simulink model "demonstrator"  (R2021a)
settings: Solver=VariableStepAuto  StartTime=0.0  StopTime=4000/3.2e6  RelTol=1e-3
values from neighbouring files (symbols this model uses):
  f_system = 64e6    (= 64000000)    [setup_demonstrator.m]
  fir_bbuf = reshape([fir_barker_13; fir_barker_13; fir_barker_13], [1, length(fir_barker_13)*3])    [setup_demonstrator.m]
  tx_data = [tx_data mbuf]    [setup_demonstrator.m]
undefined symbols (not defined in the file or in its folder): AXI4, designMultirateFIR, fsystem, Lite, xlfda_numerator
libraries: hdlBasic x533, hdlsllib x35, hdlDSPIP x21, hdlSSR x18, dspmlti4 x14, dspswit3 x8, dspsigops x5, vmcUtilities x4, hdlUtilities x4, simulink x3, dspsigattribs x2, commrandsrc3 x1
(part 9 of 10)

== system demonstrator/Receiver/Carrier Synchronisation/Generate Angle Error/Circular CORDIC/Vectoring Cell 1 ==
  x in : Inport
  y in : Inport  Port=2
  z in : Inport  Port=3
  AddSub1 : hdlBasic/AddSub  mode=Addition or Subtraction  use_carryin=off  use_carryout=off  en=off  latency=0  precision=User Defined  arith_type="Signed  (2's comp)"  n_bits=20  bin_pt=18  quantization=Truncate  overflow=Wrap  use_behavioral_HDL=on  hw_selection=Fabric  pipelined=off  use_rpm=on  XmcBlockStatus=1  maskContainerNames=tabcontainer1  block_type=addsub  block_config=sysgen:Addsub_config
  AddSub2 : hdlBasic/AddSub  mode=Addition or Subtraction  use_carryin=off  use_carryout=off  en=off  latency=0  precision=User Defined  arith_type="Signed  (2's comp)"  n_bits=15  bin_pt=12  quantization=Truncate  overflow=Wrap  use_behavioral_HDL=on  hw_selection=Fabric  pipelined=off  use_rpm=on  XmcBlockStatus=1  maskContainerNames=tabcontainer1  block_type=addsub  block_config=sysgen:Addsub_config
  AddSub3 : hdlBasic/AddSub  mode=Addition or Subtraction  use_carryin=off  use_carryout=off  en=off  latency=0  precision=User Defined  arith_type="Signed  (2's comp)"  n_bits=15  bin_pt=12  quantization=Truncate  overflow=Wrap  use_behavioral_HDL=on  hw_selection=Fabric  pipelined=off  use_rpm=on  XmcBlockStatus=1  maskContainerNames=tabcontainer1  block_type=addsub  block_config=sysgen:Addsub_config
  Constant : hdlBasic/Constant  const=atan(2^-i)  gui_display_data_type=Fixed-point  arith_type=Signed (2's comp)  n_bits=20  bin_pt=18  preci_type=Single  exp_width=8  frac_width=24  explicit_period=off  period=1  XmcBlockStatus=1  maskContainerNames=tabcontainer1  block_type=constant  block_config=sysgen:Constant_config
  Inverter : hdlBasic/Inverter  en=off  latency=0  XmcBlockStatus=1  maskContainerNames=group2  block_type=inv  block_config=sysgen:Inverter_config
  Logical : hdlBasic/Logical  logical_function=XOR  inputs=2  en=off  latency=0  precision=Full  arith_type=Unsigned  n_bits=1  bin_pt=0  align_bp=on  overflow=[]  quantization=[]  XmcBlockStatus=1  maskContainerNames=tabcontainer1  block_type=logical  block_config=sysgen:Logical_config
  Shift : hdlBasic/Shift  shift_dir=Right  shift_bits=i  en=off  latency=0  precision=User Defined  arith_type="Signed  (2's comp)"  n_bits=15  bin_pt=12  quantization=Truncate  overflow=Wrap  XmcBlockStatus=1  maskContainerNames=group2  block_type=shift  block_config=sysgen:Shift_config
  Shift1 : hdlBasic/Shift  shift_dir=Right  shift_bits=i  en=off  latency=0  precision=User Defined  arith_type="Signed  (2's comp)"  n_bits=15  bin_pt=12  quantization=Truncate  overflow=Wrap  XmcBlockStatus=1  maskContainerNames=group2  block_type=shift  block_config=sysgen:Shift_config
  Slice : hdlBasic/Slice  nbits=1  boolean_output=on  mode=Upper Bit Location + Width  bit1=0  base1=MSB of Input  bit0=0  base0=LSB of Input  XmcBlockStatus=1  maskContainerNames=group1  block_type=slice  block_config=sysgen:Slice_config
  Slice1 : hdlBasic/Slice  nbits=1  boolean_output=on  mode=Upper Bit Location + Width  bit1=0  base1=MSB of Input  bit0=0  base0=LSB of Input  XmcBlockStatus=1  maskContainerNames=group1  block_type=slice  block_config=sysgen:Slice_config
  x out : Outport  VectorParamsAs1DForOutWhenUnconnected=off
  y out : Outport  Port=2  VectorParamsAs1DForOutWhenUnconnected=off
  z out : Outport  Port=3  VectorParamsAs1DForOutWhenUnconnected=off
  wires:
  AddSub1/1 -> z out/1
  Constant/1 -> AddSub1/2
  z in/1 -> AddSub1/1
  AddSub3/1 -> y out/1
  AddSub2/1 -> x out/1
  Inverter/1 -> AddSub3/3
  Shift/1 -> AddSub3/2
  Shift1/1 -> AddSub2/2
  Logical/1 -> AddSub1/3, AddSub2/3, Inverter/1
  Slice1/1 -> Logical/2
  Slice/1 -> Logical/1
  y in/1 -> Slice1/1, Shift1/1, AddSub3/1
  x in/1 -> Slice/1, Shift/1, AddSub2/1

== system demonstrator/Receiver/Carrier Synchronisation/Generate Angle Error/Circular CORDIC/Vectoring Cell 2 ==
  x in : Inport
  y in : Inport  Port=2
  z in : Inport  Port=3
  AddSub1 : hdlBasic/AddSub  mode=Addition or Subtraction  use_carryin=off  use_carryout=off  en=off  latency=0  precision=User Defined  arith_type="Signed  (2's comp)"  n_bits=20  bin_pt=18  quantization=Truncate  overflow=Wrap  use_behavioral_HDL=on  hw_selection=Fabric  pipelined=off  use_rpm=on  XmcBlockStatus=1  maskContainerNames=tabcontainer1  block_type=addsub  block_config=sysgen:Addsub_config
  AddSub2 : hdlBasic/AddSub  mode=Addition or Subtraction  use_carryin=off  use_carryout=off  en=off  latency=0  precision=User Defined  arith_type="Signed  (2's comp)"  n_bits=15  bin_pt=12  quantization=Truncate  overflow=Wrap  use_behavioral_HDL=on  hw_selection=Fabric  pipelined=off  use_rpm=on  XmcBlockStatus=1  maskContainerNames=tabcontainer1  block_type=addsub  block_config=sysgen:Addsub_config
  AddSub3 : hdlBasic/AddSub  mode=Addition or Subtraction  use_carryin=off  use_carryout=off  en=off  latency=0  precision=User Defined  arith_type="Signed  (2's comp)"  n_bits=15  bin_pt=12  quantization=Truncate  overflow=Wrap  use_behavioral_HDL=on  hw_selection=Fabric  pipelined=off  use_rpm=on  XmcBlockStatus=1  maskContainerNames=tabcontainer1  block_type=addsub  block_config=sysgen:Addsub_config
  Constant : hdlBasic/Constant  const=atan(2^-i)  gui_display_data_type=Fixed-point  arith_type=Signed (2's comp)  n_bits=20  bin_pt=18  preci_type=Single  exp_width=8  frac_width=24  explicit_period=off  period=1  XmcBlockStatus=1  maskContainerNames=tabcontainer1  block_type=constant  block_config=sysgen:Constant_config
  Inverter : hdlBasic/Inverter  en=off  latency=0  XmcBlockStatus=1  maskContainerNames=group2  block_type=inv  block_config=sysgen:Inverter_config
  Logical : hdlBasic/Logical  logical_function=XOR  inputs=2  en=off  latency=0  precision=Full  arith_type=Unsigned  n_bits=1  bin_pt=0  align_bp=on  overflow=[]  quantization=[]  XmcBlockStatus=1  maskContainerNames=tabcontainer1  block_type=logical  block_config=sysgen:Logical_config
  Shift : hdlBasic/Shift  shift_dir=Right  shift_bits=i  en=off  latency=0  precision=User Defined  arith_type="Signed  (2's comp)"  n_bits=15  bin_pt=12  quantization=Truncate  overflow=Wrap  XmcBlockStatus=1  maskContainerNames=group2  block_type=shift  block_config=sysgen:Shift_config
  Shift1 : hdlBasic/Shift  shift_dir=Right  shift_bits=i  en=off  latency=0  precision=User Defined  arith_type="Signed  (2's comp)"  n_bits=15  bin_pt=12  quantization=Truncate  overflow=Wrap  XmcBlockStatus=1  maskContainerNames=group2  block_type=shift  block_config=sysgen:Shift_config
  Slice : hdlBasic/Slice  nbits=1  boolean_output=on  mode=Upper Bit Location + Width  bit1=0  base1=MSB of Input  bit0=0  base0=LSB of Input  XmcBlockStatus=1  maskContainerNames=group1  block_type=slice  block_config=sysgen:Slice_config
  Slice1 : hdlBasic/Slice  nbits=1  boolean_output=on  mode=Upper Bit Location + Width  bit1=0  base1=MSB of Input  bit0=0  base0=LSB of Input  XmcBlockStatus=1  maskContainerNames=group1  block_type=slice  block_config=sysgen:Slice_config
  x out : Outport  VectorParamsAs1DForOutWhenUnconnected=off
  y out : Outport  Port=2  VectorParamsAs1DForOutWhenUnconnected=off
  z out : Outport  Port=3  VectorParamsAs1DForOutWhenUnconnected=off
  wires:
  x in/1 -> AddSub2/1, Shift/1, Slice/1
  y in/1 -> AddSub3/1, Shift1/1, Slice1/1
  Slice/1 -> Logical/1
  Slice1/1 -> Logical/2
  Logical/1 -> Inverter/1, AddSub2/3, AddSub1/3
  Shift1/1 -> AddSub2/2
  Shift/1 -> AddSub3/2
  Inverter/1 -> AddSub3/3
  AddSub2/1 -> x out/1
  AddSub3/1 -> y out/1
  z in/1 -> AddSub1/1
  Constant/1 -> AddSub1/2
  AddSub1/1 -> z out/1

== system demonstrator/Receiver/Carrier Synchronisation/Generate Angle Error/Circular CORDIC/Vectoring Cell 3 ==
  x in : Inport
  y in : Inport  Port=2
  z in : Inport  Port=3
  AddSub1 : hdlBasic/AddSub  mode=Addition or Subtraction  use_carryin=off  use_carryout=off  en=off  latency=0  precision=User Defined  arith_type="Signed  (2's comp)"  n_bits=20  bin_pt=18  quantization=Truncate  overflow=Wrap  use_behavioral_HDL=on  hw_selection=Fabric  pipelined=off  use_rpm=on  XmcBlockStatus=1  maskContainerNames=tabcontainer1  block_type=addsub  block_config=sysgen:Addsub_config
  AddSub2 : hdlBasic/AddSub  mode=Addition or Subtraction  use_carryin=off  use_carryout=off  en=off  latency=0  precision=User Defined  arith_type="Signed  (2's comp)"  n_bits=15  bin_pt=12  quantization=Truncate  overflow=Wrap  use_behavioral_HDL=on  hw_selection=Fabric  pipelined=off  use_rpm=on  XmcBlockStatus=1  maskContainerNames=tabcontainer1  block_type=addsub  block_config=sysgen:Addsub_config
  AddSub3 : hdlBasic/AddSub  mode=Addition or Subtraction  use_carryin=off  use_carryout=off  en=off  latency=0  precision=User Defined  arith_type="Signed  (2's comp)"  n_bits=15  bin_pt=12  quantization=Truncate  overflow=Wrap  use_behavioral_HDL=on  hw_selection=Fabric  pipelined=off  use_rpm=on  XmcBlockStatus=1  maskContainerNames=tabcontainer1  block_type=addsub  block_config=sysgen:Addsub_config
  Constant : hdlBasic/Constant  const=atan(2^-i)  gui_display_data_type=Fixed-point  arith_type=Signed (2's comp)  n_bits=20  bin_pt=18  preci_type=Single  exp_width=8  frac_width=24  explicit_period=off  period=1  XmcBlockStatus=1  maskContainerNames=tabcontainer1  block_type=constant  block_config=sysgen:Constant_config
  Inverter : hdlBasic/Inverter  en=off  latency=0  XmcBlockStatus=1  maskContainerNames=group2  block_type=inv  block_config=sysgen:Inverter_config
  Logical : hdlBasic/Logical  logical_function=XOR  inputs=2  en=off  latency=0  precision=Full  arith_type=Unsigned  n_bits=1  bin_pt=0  align_bp=on  overflow=[]  quantization=[]  XmcBlockStatus=1  maskContainerNames=tabcontainer1  block_type=logical  block_config=sysgen:Logical_config
  Shift : hdlBasic/Shift  shift_dir=Right  shift_bits=i  en=off  latency=0  precision=User Defined  arith_type="Signed  (2's comp)"  n_bits=15  bin_pt=12  quantization=Truncate  overflow=Wrap  XmcBlockStatus=1  maskContainerNames=group2  block_type=shift  block_config=sysgen:Shift_config
  Shift1 : hdlBasic/Shift  shift_dir=Right  shift_bits=i  en=off  latency=0  precision=User Defined  arith_type="Signed  (2's comp)"  n_bits=15  bin_pt=12  quantization=Truncate  overflow=Wrap  XmcBlockStatus=1  maskContainerNames=group2  block_type=shift  block_config=sysgen:Shift_config
  Slice : hdlBasic/Slice  nbits=1  boolean_output=on  mode=Upper Bit Location + Width  bit1=0  base1=MSB of Input  bit0=0  base0=LSB of Input  XmcBlockStatus=1  maskContainerNames=group1  block_type=slice  block_config=sysgen:Slice_config
  Slice1 : hdlBasic/Slice  nbits=1  boolean_output=on  mode=Upper Bit Location + Width  bit1=0  base1=MSB of Input  bit0=0  base0=LSB of Input  XmcBlockStatus=1  maskContainerNames=group1  block_type=slice  block_config=sysgen:Slice_config
  x out : Outport  VectorParamsAs1DForOutWhenUnconnected=off
  y out : Outport  Port=2  VectorParamsAs1DForOutWhenUnconnected=off
  z out : Outport  Port=3  VectorParamsAs1DForOutWhenUnconnected=off
  wires:
  AddSub1/1 -> z out/1
  Constant/1 -> AddSub1/2
  z in/1 -> AddSub1/1
  AddSub3/1 -> y out/1
  AddSub2/1 -> x out/1
  Inverter/1 -> AddSub3/3
  Shift/1 -> AddSub3/2
  Shift1/1 -> AddSub2/2
  Logical/1 -> AddSub1/3, AddSub2/3, Inverter/1
  Slice1/1 -> Logical/2
  Slice/1 -> Logical/1
  y in/1 -> Slice1/1, Shift1/1, AddSub3/1
  x in/1 -> Slice/1, Shift/1, AddSub2/1

== system demonstrator/Receiver/Carrier Synchronisation/Generate Angle Error/Circular CORDIC/Vectoring Cell 4 ==
  x in : Inport
  y in : Inport  Port=2
  z in : Inport  Port=3
  AddSub1 : hdlBasic/AddSub  mode=Addition or Subtraction  use_carryin=off  use_carryout=off  en=off  latency=0  precision=User Defined  arith_type="Signed  (2's comp)"  n_bits=20  bin_pt=18  quantization=Truncate  overflow=Wrap  use_behavioral_HDL=on  hw_selection=Fabric  pipelined=off  use_rpm=on  XmcBlockStatus=1  maskContainerNames=tabcontainer1  block_type=addsub  block_config=sysgen:Addsub_config
  AddSub2 : hdlBasic/AddSub  mode=Addition or Subtraction  use_carryin=off  use_carryout=off  en=off  latency=0  precision=User Defined  arith_type="Signed  (2's comp)"  n_bits=15  bin_pt=12  quantization=Truncate  overflow=Wrap  use_behavioral_HDL=on  hw_selection=Fabric  pipelined=off  use_rpm=on  XmcBlockStatus=1  maskContainerNames=tabcontainer1  block_type=addsub  block_config=sysgen:Addsub_config
  AddSub3 : hdlBasic/AddSub  mode=Addition or Subtraction  use_carryin=off  use_carryout=off  en=off  latency=0  precision=User Defined  arith_type="Signed  (2's comp)"  n_bits=15  bin_pt=12  quantization=Truncate  overflow=Wrap  use_behavioral_HDL=on  hw_selection=Fabric  pipelined=off  use_rpm=on  XmcBlockStatus=1  maskContainerNames=tabcontainer1  block_type=addsub  block_config=sysgen:Addsub_config
  Constant : hdlBasic/Constant  const=atan(2^-i)  gui_display_data_type=Fixed-point  arith_type=Signed (2's comp)  n_bits=20  bin_pt=18  preci_type=Single  exp_width=8  frac_width=24  explicit_period=off  period=1  XmcBlockStatus=1  maskContainerNames=tabcontainer1  block_type=constant  block_config=sysgen:Constant_config
  Inverter : hdlBasic/Inverter  en=off  latency=0  XmcBlockStatus=1  maskContainerNames=group2  block_type=inv  block_config=sysgen:Inverter_config
  Logical : hdlBasic/Logical  logical_function=XOR  inputs=2  en=off  latency=0  precision=Full  arith_type=Unsigned  n_bits=1  bin_pt=0  align_bp=on  overflow=[]  quantization=[]  XmcBlockStatus=1  maskContainerNames=tabcontainer1  block_type=logical  block_config=sysgen:Logical_config
  Shift : hdlBasic/Shift  shift_dir=Right  shift_bits=i  en=off  latency=0  precision=User Defined  arith_type="Signed  (2's comp)"  n_bits=15  bin_pt=12  quantization=Truncate  overflow=Wrap  XmcBlockStatus=1  maskContainerNames=group2  block_type=shift  block_config=sysgen:Shift_config
  Shift1 : hdlBasic/Shift  shift_dir=Right  shift_bits=i  en=off  latency=0  precision=User Defined  arith_type="Signed  (2's comp)"  n_bits=15  bin_pt=12  quantization=Truncate  overflow=Wrap  XmcBlockStatus=1  maskContainerNames=group2  block_type=shift  block_config=sysgen:Shift_config
  Slice : hdlBasic/Slice  nbits=1  boolean_output=on  mode=Upper Bit Location + Width  bit1=0  base1=MSB of Input  bit0=0  base0=LSB of Input  XmcBlockStatus=1  maskContainerNames=group1  block_type=slice  block_config=sysgen:Slice_config
  Slice1 : hdlBasic/Slice  nbits=1  boolean_output=on  mode=Upper Bit Location + Width  bit1=0  base1=MSB of Input  bit0=0  base0=LSB of Input  XmcBlockStatus=1  maskContainerNames=group1  block_type=slice  block_config=sysgen:Slice_config
  x out : Outport  VectorParamsAs1DForOutWhenUnconnected=off
  y out : Outport  Port=2  VectorParamsAs1DForOutWhenUnconnected=off
  z out : Outport  Port=3  VectorParamsAs1DForOutWhenUnconnected=off
  wires:
  x in/1 -> AddSub2/1, Shift/1, Slice/1
  y in/1 -> AddSub3/1, Shift1/1, Slice1/1
  Slice/1 -> Logical/1
  Slice1/1 -> Logical/2
  Logical/1 -> Inverter/1, AddSub2/3, AddSub1/3
  Shift1/1 -> AddSub2/2
  Shift/1 -> AddSub3/2
  Inverter/1 -> AddSub3/3
  AddSub2/1 -> x out/1
  AddSub3/1 -> y out/1
  z in/1 -> AddSub1/1
  Constant/1 -> AddSub1/2
  AddSub1/1 -> z out/1

== system demonstrator/Receiver/Carrier Synchronisation/Generate Angle Error/Circular CORDIC/Vectoring Cell 5 ==
  x in : Inport
  y in : Inport  Port=2
  z in : Inport  Port=3
  AddSub1 : hdlBasic/AddSub  mode=Addition or Subtraction  use_carryin=off  use_carryout=off  en=off  latency=0  precision=User Defined  arith_type="Signed  (2's comp)"  n_bits=20  bin_pt=18  quantization=Truncate  overflow=Wrap  use_behavioral_HDL=on  hw_selection=Fabric  pipelined=off  use_rpm=on  XmcBlockStatus=1  maskContainerNames=tabcontainer1  block_type=addsub  block_config=sysgen:Addsub_config
  AddSub2 : hdlBasic/AddSub  mode=Addition or Subtraction  use_carryin=off  use_carryout=off  en=off  latency=0  precision=User Defined  arith_type="Signed  (2's comp)"  n_bits=15  bin_pt=12  quantization=Truncate  overflow=Wrap  use_behavioral_HDL=on  hw_selection=Fabric  pipelined=off  use_rpm=on  XmcBlockStatus=1  maskContainerNames=tabcontainer1  block_type=addsub  block_config=sysgen:Addsub_config
  AddSub3 : hdlBasic/AddSub  mode=Addition or Subtraction  use_carryin=off  use_carryout=off  en=off  latency=0  precision=User Defined  arith_type="Signed  (2's comp)"  n_bits=15  bin_pt=12  quantization=Truncate  overflow=Wrap  use_behavioral_HDL=on  hw_selection=Fabric  pipelined=off  use_rpm=on  XmcBlockStatus=1  maskContainerNames=tabcontainer1  block_type=addsub  block_config=sysgen:Addsub_config
  Constant : hdlBasic/Constant  const=atan(2^-i)  gui_display_data_type=Fixed-point  arith_type=Signed (2's comp)  n_bits=20  bin_pt=18  preci_type=Single  exp_width=8  frac_width=24  explicit_period=off  period=1  XmcBlockStatus=1  maskContainerNames=tabcontainer1  block_type=constant  block_config=sysgen:Constant_config
  Inverter : hdlBasic/Inverter  en=off  latency=0  XmcBlockStatus=1  maskContainerNames=group2  block_type=inv  block_config=sysgen:Inverter_config
  Logical : hdlBasic/Logical  logical_function=XOR  inputs=2  en=off  latency=0  precision=Full  arith_type=Unsigned  n_bits=1  bin_pt=0  align_bp=on  overflow=[]  quantization=[]  XmcBlockStatus=1  maskContainerNames=tabcontainer1  block_type=logical  block_config=sysgen:Logical_config
  Shift : hdlBasic/Shift  shift_dir=Right  shift_bits=i  en=off  latency=0  precision=User Defined  arith_type="Signed  (2's comp)"  n_bits=15  bin_pt=12  quantization=Truncate  overflow=Wrap  XmcBlockStatus=1  maskContainerNames=group2  block_type=shift  block_config=sysgen:Shift_config
  Shift1 : hdlBasic/Shift  shift_dir=Right  shift_bits=i  en=off  latency=0  precision=User Defined  arith_type="Signed  (2's comp)"  n_bits=15  bin_pt=12  quantization=Truncate  overflow=Wrap  XmcBlockStatus=1  maskContainerNames=group2  block_type=shift  block_config=sysgen:Shift_config
  Slice : hdlBasic/Slice  nbits=1  boolean_output=on  mode=Upper Bit Location + Width  bit1=0  base1=MSB of Input  bit0=0  base0=LSB of Input  XmcBlockStatus=1  maskContainerNames=group1  block_type=slice  block_config=sysgen:Slice_config
  Slice1 : hdlBasic/Slice  nbits=1  boolean_output=on  mode=Upper Bit Location + Width  bit1=0  base1=MSB of Input  bit0=0  base0=LSB of Input  XmcBlockStatus=1  maskContainerNames=group1  block_type=slice  block_config=sysgen:Slice_config
  x out : Outport  VectorParamsAs1DForOutWhenUnconnected=off
  y out : Outport  Port=2  VectorParamsAs1DForOutWhenUnconnected=off
  z out : Outport  Port=3  VectorParamsAs1DForOutWhenUnconnected=off
  wires:
  AddSub1/1 -> z out/1
  Constant/1 -> AddSub1/2
  z in/1 -> AddSub1/1
  AddSub3/1 -> y out/1
  AddSub2/1 -> x out/1
  Inverter/1 -> AddSub3/3
  Shift/1 -> AddSub3/2
  Shift1/1 -> AddSub2/2
  Logical/1 -> AddSub1/3, AddSub2/3, Inverter/1
  Slice1/1 -> Logical/2
  Slice/1 -> Logical/1
  y in/1 -> Slice1/1, Shift1/1, AddSub3/1
  x in/1 -> Slice/1, Shift/1, AddSub2/1

== system demonstrator/Receiver/Carrier Synchronisation/Generate Angle Error/Circular CORDIC/Vectoring Cell 6 ==
  x in : Inport
  y in : Inport  Port=2
  z in : Inport  Port=3
  AddSub1 : hdlBasic/AddSub  mode=Addition or Subtraction  use_carryin=off  use_carryout=off  en=off  latency=0  precision=User Defined  arith_type="Signed  (2's comp)"  n_bits=20  bin_pt=18  quantization=Truncate  overflow=Wrap  use_behavioral_HDL=on  hw_selection=Fabric  pipelined=off  use_rpm=on  XmcBlockStatus=1  maskContainerNames=tabcontainer1  block_type=addsub  block_config=sysgen:Addsub_config
  AddSub2 : hdlBasic/AddSub  mode=Addition or Subtraction  use_carryin=off  use_carryout=off  en=off  latency=0  precision=User Defined  arith_type="Signed  (2's comp)"  n_bits=15  bin_pt=12  quantization=Truncate  overflow=Wrap  use_behavioral_HDL=on  hw_selection=Fabric  pipelined=off  use_rpm=on  XmcBlockStatus=1  maskContainerNames=tabcontainer1  block_type=addsub  block_config=sysgen:Addsub_config
  AddSub3 : hdlBasic/AddSub  mode=Addition or Subtraction  use_carryin=off  use_carryout=off  en=off  latency=0  precision=User Defined  arith_type="Signed  (2's comp)"  n_bits=15  bin_pt=12  quantization=Truncate  overflow=Wrap  use_behavioral_HDL=on  hw_selection=Fabric  pipelined=off  use_rpm=on  XmcBlockStatus=1  maskContainerNames=tabcontainer1  block_type=addsub  block_config=sysgen:Addsub_config
  Constant : hdlBasic/Constant  const=atan(2^-i)  gui_display_data_type=Fixed-point  arith_type=Signed (2's comp)  n_bits=20  bin_pt=18  preci_type=Single  exp_width=8  frac_width=24  explicit_period=off  period=1  XmcBlockStatus=1  maskContainerNames=tabcontainer1  block_type=constant  block_config=sysgen:Constant_config
  Inverter : hdlBasic/Inverter  en=off  latency=0  XmcBlockStatus=1  maskContainerNames=group2  block_type=inv  block_config=sysgen:Inverter_config
  Logical : hdlBasic/Logical  logical_function=XOR  inputs=2  en=off  latency=0  precision=Full  arith_type=Unsigned  n_bits=1  bin_pt=0  align_bp=on  overflow=[]  quantization=[]  XmcBlockStatus=1  maskContainerNames=tabcontainer1  block_type=logical  block_config=sysgen:Logical_config
  Shift : hdlBasic/Shift  shift_dir=Right  shift_bits=i  en=off  latency=0  precision=User Defined  arith_type="Signed  (2's comp)"  n_bits=15  bin_pt=12  quantization=Truncate  overflow=Wrap  XmcBlockStatus=1  maskContainerNames=group2  block_type=shift  block_config=sysgen:Shift_config
  Shift1 : hdlBasic/Shift  shift_dir=Right  shift_bits=i  en=off  latency=0  precision=User Defined  arith_type="Signed  (2's comp)"  n_bits=15  bin_pt=12  quantization=Truncate  overflow=Wrap  XmcBlockStatus=1  maskContainerNames=group2  block_type=shift  block_config=sysgen:Shift_config
  Slice : hdlBasic/Slice  nbits=1  boolean_output=on  mode=Upper Bit Location + Width  bit1=0  base1=MSB of Input  bit0=0  base0=LSB of Input  XmcBlockStatus=1  maskContainerNames=group1  block_type=slice  block_config=sysgen:Slice_config
  Slice1 : hdlBasic/Slice  nbits=1  boolean_output=on  mode=Upper Bit Location + Width  bit1=0  base1=MSB of Input  bit0=0  base0=LSB of Input  XmcBlockStatus=1  maskContainerNames=group1  block_type=slice  block_config=sysgen:Slice_config
  x out : Outport  VectorParamsAs1DForOutWhenUnconnected=off
  y out : Outport  Port=2  VectorParamsAs1DForOutWhenUnconnected=off
  z out : Outport  Port=3  VectorParamsAs1DForOutWhenUnconnected=off
  wires:
  x in/1 -> AddSub2/1, Shift/1, Slice/1
  y in/1 -> AddSub3/1, Shift1/1, Slice1/1
  Slice/1 -> Logical/1
  Slice1/1 -> Logical/2
  Logical/1 -> Inverter/1, AddSub2/3, AddSub1/3
  Shift1/1 -> AddSub2/2
  Shift/1 -> AddSub3/2
  Inverter/1 -> AddSub3/3
  AddSub2/1 -> x out/1
  AddSub3/1 -> y out/1
  z in/1 -> AddSub1/1
  Constant/1 -> AddSub1/2
  AddSub1/1 -> z out/1

== system demonstrator/Receiver/Carrier Synchronisation/Generate Angle Error/Circular CORDIC/Vectoring Cell 7 ==
  x in : Inport
  y in : Inport  Port=2
  z in : Inport  Port=3
  AddSub1 : hdlBasic/AddSub  mode=Addition or Subtraction  use_carryin=off  use_carryout=off  en=off  latency=0  precision=User Defined  arith_type="Signed  (2's comp)"  n_bits=20  bin_pt=18  quantization=Truncate  overflow=Wrap  use_behavioral_HDL=on  hw_selection=Fabric  pipelined=off  use_rpm=on  XmcBlockStatus=1  maskContainerNames=tabcontainer1  block_type=addsub  block_config=sysgen:Addsub_config
  AddSub2 : hdlBasic/AddSub  mode=Addition or Subtraction  use_carryin=off  use_carryout=off  en=off  latency=0  precision=User Defined  arith_type="Signed  (2's comp)"  n_bits=15  bin_pt=12  quantization=Truncate  overflow=Wrap  use_behavioral_HDL=on  hw_selection=Fabric  pipelined=off  use_rpm=on  XmcBlockStatus=1  maskContainerNames=tabcontainer1  block_type=addsub  block_config=sysgen:Addsub_config
  AddSub3 : hdlBasic/AddSub  mode=Addition or Subtraction  use_carryin=off  use_carryout=off  en=off  latency=0  precision=User Defined  arith_type="Signed  (2's comp)"  n_bits=15  bin_pt=12  quantization=Truncate  overflow=Wrap  use_behavioral_HDL=on  hw_selection=Fabric  pipelined=off  use_rpm=on  XmcBlockStatus=1  maskContainerNames=tabcontainer1  block_type=addsub  block_config=sysgen:Addsub_config
  Constant : hdlBasic/Constant  const=atan(2^-i)  gui_display_data_type=Fixed-point  arith_type=Signed (2's comp)  n_bits=20  bin_pt=18  preci_type=Single  exp_width=8  frac_width=24  explicit_period=off  period=1  XmcBlockStatus=1  maskContainerNames=tabcontainer1  block_type=constant  block_config=sysgen:Constant_config
  Inverter : hdlBasic/Inverter  en=off  latency=0  XmcBlockStatus=1  maskContainerNames=group2  block_type=inv  block_config=sysgen:Inverter_config
  Logical : hdlBasic/Logical  logical_function=XOR  inputs=2  en=off  latency=0  precision=Full  arith_type=Unsigned  n_bits=1  bin_pt=0  align_bp=on  overflow=[]  quantization=[]  XmcBlockStatus=1  maskContainerNames=tabcontainer1  block_type=logical  block_config=sysgen:Logical_config
  Shift : hdlBasic/Shift  shift_dir=Right  shift_bits=i  en=off  latency=0  precision=User Defined  arith_type="Signed  (2's comp)"  n_bits=15  bin_pt=12  quantization=Truncate  overflow=Wrap  XmcBlockStatus=1  maskContainerNames=group2  block_type=shift  block_config=sysgen:Shift_config
  Shift1 : hdlBasic/Shift  shift_dir=Right  shift_bits=i  en=off  latency=0  precision=User Defined  arith_type="Signed  (2's comp)"  n_bits=15  bin_pt=12  quantization=Truncate  overflow=Wrap  XmcBlockStatus=1  maskContainerNames=group2  block_type=shift  block_config=sysgen:Shift_config
  Slice : hdlBasic/Slice  nbits=1  boolean_output=on  mode=Upper Bit Location + Width  bit1=0  base1=MSB of Input  bit0=0  base0=LSB of Input  XmcBlockStatus=1  maskContainerNames=group1  block_type=slice  block_config=sysgen:Slice_config
  Slice1 : hdlBasic/Slice  nbits=1  boolean_output=on  mode=Upper Bit Location + Width  bit1=0  base1=MSB of Input  bit0=0  base0=LSB of Input  XmcBlockStatus=1  maskContainerNames=group1  block_type=slice  block_config=sysgen:Slice_config
  x out : Outport  VectorParamsAs1DForOutWhenUnconnected=off
  y out : Outport  Port=2  VectorParamsAs1DForOutWhenUnconnected=off
  z out : Outport  Port=3  VectorParamsAs1DForOutWhenUnconnected=off
  wires:
  AddSub1/1 -> z out/1
  Constant/1 -> AddSub1/2
  z in/1 -> AddSub1/1
  AddSub3/1 -> y out/1
  AddSub2/1 -> x out/1
  Inverter/1 -> AddSub3/3
  Shift/1 -> AddSub3/2
  Shift1/1 -> AddSub2/2
  Logical/1 -> AddSub1/3, AddSub2/3, Inverter/1
  Slice1/1 -> Logical/2
  Slice/1 -> Logical/1
  y in/1 -> Slice1/1, Shift1/1, AddSub3/1
  x in/1 -> Slice/1, Shift/1, AddSub2/1

== system demonstrator/FINNadapter/Decimation/Stimulus and Channel/Channel/RF-ADC/Decimation Filter ==
  Data In : Inport
  FIR 0 : dspmlti4/FIR Decimation  Commented=through  FilterSource=Filter object  h=designMultirateFIR(1,2)  D=2  filtStruct=Direct form  FilterObject=fir0  InputProcessing=Columns as channels (frame based)  framing=Allow multirate processing  inputOffset=0  outputBufInitCond=0  roundingMode=Floor  overflowMode=off  firstCoeffDataTypeStr=Inherit: Same word length as input  firstCoeffMin=[]  firstCoeffMax=[]  firstCoeffLastDataTypeStr=Inherit: Same word length as input  outputDataTypeStr=Inherit: Same as accumulator  outputMin=[]  outputMax=[]  outputLastDataTypeStr=Inherit: Same as accumulator
  FIR 1 : dspmlti4/FIR Decimation  Commented=through  FilterSource=Filter object  h=designMultirateFIR(1,2)  D=2  filtStruct=Direct form  FilterObject=fir1  InputProcessing=Columns as channels (frame based)  framing=Allow multirate processing  inputOffset=0  outputBufInitCond=0  roundingMode=Floor  overflowMode=off  firstCoeffDataTypeStr=Inherit: Same word length as input  firstCoeffMin=[]  firstCoeffMax=[]  firstCoeffLastDataTypeStr=Inherit: Same word length as input  outputDataTypeStr=Inherit: Same as accumulator  outputMin=[]  outputMax=[]  outputLastDataTypeStr=Inherit: Same as accumulator
  FIR 2 : dspmlti4/FIR Decimation  FilterSource=Filter object  h=designMultirateFIR(1,2)  D=2  filtStruct=Direct form  FilterObject=fir2  InputProcessing=Columns as channels (frame based)  framing=Allow multirate processing  inputOffset=0  outputBufInitCond=0  roundingMode=Floor  overflowMode=off  firstCoeffDataTypeStr=Inherit: Same word length as input  firstCoeffMin=[]  firstCoeffMax=[]  firstCoeffLastDataTypeStr=Inherit: Same word length as input  outputDataTypeStr=Inherit: Same as accumulator  outputMin=[]  outputMax=[]  outputLastDataTypeStr=Inherit: Same as accumulator
  Data Out : Outport  VectorParamsAs1DForOutWhenUnconnected=off
  wires:
  FIR 1/1 -> FIR 2/1
  FIR 0/1 -> FIR 1/1
  Data In/1 -> FIR 0/1
  FIR 2/1 -> Data Out/1

== system demonstrator/FINNadapter/Decimation/Stimulus and Channel/Channel/RF-ADC/NCO and Mixer ==
  Data In : Inport
  Constant1 : Constant  Value=m  OutDataTypeStr=fixdt(0,2,0)  SampleTime=-1
  Data Type Conversion : DataTypeConversion  OutDataTypeStr=fixdt(1,16,15)
  Multiport Switch1 : MultiPortSwitch  DataPortOrder=Zero-based contiguous  zeroidx=on
  RF-ADC Coarse Mixer : Subsystem
  RF-ADC Fine Mixer : Subsystem
  Real-Imag to Complex : RealImagToComplex
  Data Out : Outport  VectorParamsAs1DForOutWhenUnconnected=off
  wires:
  Multiport Switch1/1 -> Data Out/1
  RF-ADC Fine Mixer/1(Data Out) -> Multiport Switch1/4
  Real-Imag to Complex/1 -> Data Type Conversion/1
  RF-ADC Coarse Mixer/1(Data Out) -> Multiport Switch1/3
  Data In/1 -> Real-Imag to Complex/1, RF-ADC Coarse Mixer/1(Data In), RF-ADC Fine Mixer/1(Data In), Real-Imag to Complex/2
  Constant1/1 -> Multiport Switch1/1
  Data Type Conversion/1 -> Multiport Switch1/2

== system demonstrator/FINNadapter/Decimation/Stimulus and Channel/Channel/RF-ADC/RF-ADC ==
  Data In : Inport
  Buffer : Buffer  N=ssr  OutputFrames=off
  Data Type Conversion : DataTypeConversion  OutDataTypeStr=fixdt(1,12,11)  SaturateOnIntegerOverflow=on
  Rate Transition : RateTransition  OutPortSampleTime=1/fs
  Data Out : Outport  VectorParamsAs1DForOutWhenUnconnected=off
  wires:
  Rate Transition/1 -> Data Type Conversion/1
  Data In/1 -> Rate Transition/1
  Data Type Conversion/1 -> Buffer/1
  Buffer/1 -> Data Out/1

== system demonstrator/FINNadapter/Decimation/Stimulus and Channel/Channel/RF-ADC/SSR Converter RF-ADC ==
  Real In : Inport
  Imag In : Inport  Port=2
  Constant : Constant  OutDataTypeStr=boolean  SampleTime=-1
  Convert 2-D to 1-D : dspsigattribs/Convert 2-D to 1-D
      settings: SourceProductBaseCode=DS
  Convert 2-D to 1-D1 : dspsigattribs/Convert 2-D to 1-D
      settings: SourceProductBaseCode=DS
  Vector to SSR Imag : Subsystem  mask{N=8, hN=8}
      mask prompts: N "Samples per clock cycle:"
      mask init:
      | if ~isequal(get_param(gcb, 'N'), get_param(gcb, 'hN'))
      |     % Delete all blocks except input and output ports
      |     delete_block(setxor(setdiff(...
      |         find_system(gcb,'LookUnderMasks','on'),...
      |         {[gcb, '/Vector'], [gcb, '/SSR']}), gcb));
      | 
      |     % Delete all wires
      |     delete_line(find_system(gcb, 'FindAll', 'on', 'LookUnderMasks',...
      |         'on', 'SearchDepth', 3, 'Type', 'line', 'Connected', 'off'));
      | 
      |     % Add the bit concatenation block
      |     add_block('hdlsllib/Logic and Bit Operations/Bit Concat',...
      |         [gcb, '/Bit Concat'],...
      |         'Position', [155 55 205 330]);
      |     set_param([gcb, '/Bit Concat'], 'numInputs', num2str(N));
      | 
      |     % Add wire to output
      |     add_line(gcb, 'Bit Concat/1', 'SSR/1');
      | 
      |     % Add selector blocks and connect wires
      |     for i = 0:N-1
      |         add_block('simulink/Signal Routing/Selector',...
      |             [gcb, '/Selector', num2str(i)],...
      |             'Position', [0 82+i*90 45 128+i*90]);
      |         set_param([gcb, '/Selector', num2str(i)], 'InputPortWidth', num2str(N), 'IndexParamArray', {num2str(N-i)});
      |         add_line(gcb, 'Vector/1', ['Selector', num2str(i), '/1'],...
      |             'autorouting', 'on');
      |         add_line(gcb, ['Selector', num2str(i), '/1'],...
      |             ['Bit Concat/', num2str(i+1)],...
      |             'autorouting', 'on');
      |     end
      |     
      |     % Set the hidden attribute to prevent unnecessary changes in
      |     % architecture while generating HDL Code.
      |     set_param(gcb, 'hN', get_param(gcb, 'N'));
      | end
      mask DialogControl DescGroupVar Prompt: Vector to SSR
      mask DialogControl DescTextVar Prompt: Convert a vector of inputs into SSR format.
  Vector to SSR Real : Subsystem  mask{N=8, hN=8}
      mask prompts: N "Samples per clock cycle:"
      mask init: same as demonstrator/FINNadapter/Decimation/Stimulus and Channel/Channel/RF-ADC/SSR Converter RF-ADC/Vector to SSR Imag
      mask DialogControl DescGroupVar Prompt: Vector to SSR
      mask DialogControl DescTextVar Prompt: Convert a vector of inputs into SSR format.
  Valid Real : Outport
  Valid Imag : Outport  Port=2
  Real Out : Outport  Port=3
  Imag Out : Outport  Port=4
  wires:
  Real In/1 -> Convert 2-D to 1-D/1
  Imag In/1 -> Convert 2-D to 1-D1/1
  Convert 2-D to 1-D/1 -> Vector to SSR Real/1(Vector)
  Convert 2-D to 1-D1/1 -> Vector to SSR Imag/1(Vector)
  Vector to SSR Real/1(SSR) -> Real Out/1
  Vector to SSR Imag/1(SSR) -> Imag Out/1
  Constant/1 -> Valid Imag/1, Valid Real/1

== system demonstrator/FINNadapter/Decimation/Stimulus and Channel/Channel/RF-DAC/Interpolation Filter ==
  Data In : Inport
  FIR 0 : dspmlti4/FIR Interpolation  Commented=through  FilterSource=Filter object  PrivateCoeffs=0  h=designMultirateFIR(3,1)  L=2  FilterObject=fir0  InputProcessing=Columns as channels (frame based)  framing=Allow multirate processing  outputBufInitCond=0  roundingMode=Floor  overflowMode=off  firstCoeffDataTypeStr=Inherit: Same word length as input  firstCoeffMin=[]  firstCoeffMax=[]  firstCoeffLastDataTypeStr=Inherit: Same word length as input  outputDataTypeStr=Inherit: Same as accumulator  outputMin=[]  outputMax=[]  outputLastDataTypeStr=Inherit: Same as accumulator
  FIR 1 : dspmlti4/FIR Interpolation  FilterSource=Filter object  PrivateCoeffs=0  h=designMultirateFIR(3,1)  L=2  FilterObject=fir1  InputProcessing=Columns as channels (frame based)  framing=Allow multirate processing  outputBufInitCond=0  roundingMode=Floor  overflowMode=off  firstCoeffDataTypeStr=Inherit: Same word length as input  firstCoeffMin=[]  firstCoeffMax=[]  firstCoeffLastDataTypeStr=Inherit: Same word length as input  outputDataTypeStr=Inherit: Same as accumulator  outputMin=[]  outputMax=[]  outputLastDataTypeStr=Inherit: Same as accumulator
  FIR 2 : dspmlti4/FIR Interpolation  FilterSource=Filter object  PrivateCoeffs=0  h=designMultirateFIR(3,1)  L=2  FilterObject=fir2  InputProcessing=Columns as channels (frame based)  framing=Allow multirate processing  outputBufInitCond=0  roundingMode=Floor  overflowMode=off  firstCoeffDataTypeStr=Inherit: Same word length as input  firstCoeffMin=[]  firstCoeffMax=[]  firstCoeffLastDataTypeStr=Inherit: Same word length as input  outputDataTypeStr=Inherit: Same as accumulator  outputMin=[]  outputMax=[]  outputLastDataTypeStr=Inherit: Same as accumulator
  Data Out : Outport  VectorParamsAs1DForOutWhenUnconnected=off
  wires:
  FIR 2/1 -> FIR 1/1
  Data In/1 -> FIR 2/1
  FIR 0/1 -> Data Out/1
  FIR 1/1 -> FIR 0/1

== system demonstrator/FINNadapter/Decimation/Stimulus and Channel/Channel/RF-DAC/NCO and Mixer ==
  Data In : Inport
  Complex to Real-Imag : ComplexToRealImag
  Constant1 : Constant  Value=m  OutDataTypeStr=fixdt(0,2,0)  SampleTime=-1
  Multiport Switch1 : MultiPortSwitch  DataPortOrder=Zero-based contiguous  zeroidx=on
  RF-DAC Coarse Mixer : Subsystem
  RF-DAC Fine Mixer : Subsystem
  Terminator : Terminator
  Data Out : Outport  VectorParamsAs1DForOutWhenUnconnected=off
  wires:
  RF-DAC Coarse Mixer/1(Data Out) -> Multiport Switch1/3
  Constant1/1 -> Multiport Switch1/1
  Data In/1 -> Complex to Real-Imag/1, RF-DAC Coarse Mixer/1(Data In), RF-DAC Fine Mixer/1(Data In)
  Multiport Switch1/1 -> Data Out/1
  RF-DAC Fine Mixer/1(Data Out) -> Multiport Switch1/4
  Complex to Real-Imag/1 -> Multiport Switch1/2
  Complex to Real-Imag/2 -> Terminator/1

== system demonstrator/FINNadapter/Decimation/Stimulus and Channel/Channel/RF-DAC/RF-DAC ==
  Data In : Inport
  Cast To Double : DataTypeConversion  OutDataTypeStr=double
  Rate Transition : RateTransition  OutPortSampleTime=0
  Unbuffer : Unbuffer
  Data Out : Outport  VectorParamsAs1DForOutWhenUnconnected=off
  wires:
  Cast To Double/1 -> Rate Transition/1
  Unbuffer/1 -> Cast To Double/1
  Data In/1 -> Unbuffer/1
  Rate Transition/1 -> Data Out/1

== system demonstrator/FINNadapter/Decimation/Stimulus and Channel/Channel/RF-DAC/SSR Converter RF-DAC ==
  Valid : Inport
  Data : Inport  Port=2
  Bit Slice Imag1 : hdlsllib/Logic and Bit Operations/Bit Slice  lidx=31  ridx=16
      settings: SourceProductBaseCode=SL
  Bit Slice Real1 : hdlsllib/Logic and Bit Operations/Bit Slice  lidx=15  ridx=0
      settings: SourceProductBaseCode=SL
  Data Type Conversion : DataTypeConversion  OutDataTypeStr=fixdt(1,16,15)  ConvertRealWorld=Stored Integer (SI)
  Real-Imag to Complex1 : RealImagToComplex
  SSR to Vector Low : Subsystem  mask{N=ssr, w=32, hN=ssr, hw=32}
      mask prompts: N "Samples per clock cycle:"; w "Wordlength:"
      mask init: same as demonstrator/FINNadapter/Decimation/Convert for Analysis/SSR to Vector Imag
      mask DialogControl DescGroupVar Prompt: SSR to Vector
      mask DialogControl DescTextVar Prompt: Convert the SSR vector format based on the wordlength and expected number of samples per clock cycle.
  Terminator : Terminator
  Data Out : Outport
  wires:
  Data/1 -> SSR to Vector Low/1(SSR)
  Bit Slice Imag1/1 -> Real-Imag to Complex1/2
  Bit Slice Real1/1 -> Real-Imag to Complex1/1
  SSR to Vector Low/1(Vector) -> Bit Slice Imag1/1, Bit Slice Real1/1
  Data Type Conversion/1 -> Data Out/1
  Valid/1 -> Terminator/1
  Real-Imag to Complex1/1 -> Data Type Conversion/1

== system demonstrator/FINNadapter/Decimation/Stimulus and Channel/Transmitter/Transmitter/Vector to SSR Low ==
  Vector : Inport
  Bit Concat : hdlsllib/Logic and Bit Operations/Bit Concat  numInputs=4
  Selector0 : Selector  InputPortWidth=4  IndexOptions=Index vector (dialog)  Indices=4  OutputSizes=1
  Selector1 : Selector  InputPortWidth=4  IndexOptions=Index vector (dialog)  Indices=3  OutputSizes=1
  Selector2 : Selector  InputPortWidth=4  IndexOptions=Index vector (dialog)  Indices=2  OutputSizes=1
  Selector3 : Selector  InputPortWidth=4  IndexOptions=Index vector (dialog)  Indices=1  OutputSizes=1
  SSR : Outport
  wires:
  Bit Concat/1 -> SSR/1
  Vector/1 -> Selector0/1, Selector1/1, Selector2/1, Selector3/1
  Selector0/1 -> Bit Concat/1
  Selector1/1 -> Bit Concat/2
  Selector2/1 -> Bit Concat/3
  Selector3/1 -> Bit Concat/4

== system demonstrator/FINNadapter/Decimation/Stimulus and Channel/Channel/RF-ADC/NCO and Mixer/RF-ADC Coarse Mixer ==
  Data In : Inport
  Constant : Constant  Value=mc  OutDataTypeStr=fixdt(0,2,0)  SampleTime=-1
  Data Type Conversion : DataTypeConversion  OutDataTypeStr=fixdt(1,16,15)
  Multiport Switch1 : MultiPortSwitch  DataPortOrder=Zero-based contiguous  zeroidx=on
  Negate : Subsystem
  fs_2 : Subsystem
  fs_4 : Subsystem
  Data Out : Outport  VectorParamsAs1DForOutWhenUnconnected=off
  wires:
  Multiport Switch1/1 -> Data Type Conversion/1
  fs_2/1(Data Out) -> Multiport Switch1/2
  Constant/1 -> Multiport Switch1/1
  Data In/1 -> fs_4/1(Data In), fs_2/1(Data In)
  Negate/1(Data Out) -> Multiport Switch1/4
  fs_4/1(Data Out) -> Negate/1(Data In), Multiport Switch1/3
  Data Type Conversion/1 -> Data Out/1

== system demonstrator/FINNadapter/Decimation/Stimulus and Channel/Channel/RF-ADC/NCO and Mixer/RF-ADC Fine Mixer ==
  Data In : Inport
  Complex to Real-Imag : ComplexToRealImag
  Constant : Constant  Value=0  SampleTime=-1
  Multiport Switch : MultiPortSwitch  DataPortOrder=Zero-based contiguous  Inputs=2  zeroidx=on
  NCO : dspsigops/NCO  AccIncSrc=Specify via dialog  AccInc=fix((((fc*1e9)*(2^18))/(fs))*2^30)  PhaseOffsetSrc=Specify via dialog  PhaseOffset=fix((((2^18)*fph)/(2*pi))*2^30)  AccumWL=48  HasDither=off  DitherWL=4  PNgeneratorLength=19  HasPhaseQuantizer=on  TableDepth=18  HasOutputPhaseError=off  Formula=Sine and cosine  DataType=Binary point scaling  OutputWL=16  OutputFL=15  CompMethod=Table lookup (no interpolation)  SampleTime=1/(fs)  SamplesPerFrame=ssr  OutputFrames=off
      settings: SourceProductBaseCode=DS
  Product : Product  OutDataTypeStr=fixdt(1,16,15)
  Product1 : Product  OutDataTypeStr=fixdt(1,16,15)
  Real-Imag to Complex : RealImagToComplex
  Real-Imag to Complex1 : RealImagToComplex
  Shift Arithmetic : ArithShift  BitShiftNumber=1  BitShiftDirection=Right
  Shift Arithmetic1 : ArithShift  BitShiftNumber=1  BitShiftDirection=Right
  Data Out : Outport  VectorParamsAs1DForOutWhenUnconnected=off
  wires:
  Data In/1 -> Product1/1, Product/1
  Constant/1 -> Multiport Switch/1
  Multiport Switch/1 -> Data Out/1
  Complex to Real-Imag/2 -> Shift Arithmetic/1
  Complex to Real-Imag/1 -> Shift Arithmetic1/1
  Shift Arithmetic1/1 -> Real-Imag to Complex1/1
  Shift Arithmetic/1 -> Real-Imag to Complex1/2
  Real-Imag to Complex1/1 -> Multiport Switch/3
  NCO/1 -> Product/2
  NCO/2 -> Product1/2
  Real-Imag to Complex/1 -> Multiport Switch/2, Complex to Real-Imag/1
  Product1/1 -> Real-Imag to Complex/1
  Product/1 -> Real-Imag to Complex/2

== system demonstrator/FINNadapter/Decimation/Stimulus and Channel/Channel/RF-ADC/SSR Converter RF-ADC/Vector to SSR Imag ==
  Vector : Inport
  Bit Concat : hdlsllib/Logic and Bit Operations/Bit Concat  numInputs=8
  Selector0 : Selector  InputPortWidth=8  IndexOptions=Index vector (dialog)  Indices=8  OutputSizes=1
  Selector1 : Selector  InputPortWidth=8  IndexOptions=Index vector (dialog)  Indices=7  OutputSizes=1
  Selector2 : Selector  InputPortWidth=8  IndexOptions=Index vector (dialog)  Indices=6  OutputSizes=1
  Selector3 : Selector  InputPortWidth=8  IndexOptions=Index vector (dialog)  Indices=5  OutputSizes=1
  Selector4 : Selector  InputPortWidth=8  IndexOptions=Index vector (dialog)  Indices=4  OutputSizes=1
  Selector5 : Selector  InputPortWidth=8  IndexOptions=Index vector (dialog)  Indices=3  OutputSizes=1
  Selector6 : Selector  InputPortWidth=8  IndexOptions=Index vector (dialog)  Indices=2  OutputSizes=1
  Selector7 : Selector  InputPortWidth=8  IndexOptions=Index vector (dialog)  Indices=1  OutputSizes=1
  SSR : Outport
  wires:
  Bit Concat/1 -> SSR/1
  Vector/1 -> Selector0/1, Selector1/1, Selector2/1, Selector3/1, Selector4/1, Selector5/1, Selector6/1, Selector7/1
  Selector0/1 -> Bit Concat/1
  Selector1/1 -> Bit Concat/2
  Selector2/1 -> Bit Concat/3
  Selector3/1 -> Bit Concat/4
  Selector4/1 -> Bit Concat/5
  Selector5/1 -> Bit Concat/6
  Selector6/1 -> Bit Concat/7
  Selector7/1 -> Bit Concat/8

== system demonstrator/FINNadapter/Decimation/Stimulus and Channel/Channel/RF-ADC/SSR Converter RF-ADC/Vector to SSR Real ==
  Vector : Inport
  Bit Concat : hdlsllib/Logic and Bit Operations/Bit Concat  numInputs=8
  Selector0 : Selector  InputPortWidth=8  IndexOptions=Index vector (dialog)  Indices=8  OutputSizes=1
  Selector1 : Selector  InputPortWidth=8  IndexOptions=Index vector (dialog)  Indices=7  OutputSizes=1
  Selector2 : Selector  InputPortWidth=8  IndexOptions=Index vector (dialog)  Indices=6  OutputSizes=1
  Selector3 : Selector  InputPortWidth=8  IndexOptions=Index vector (dialog)  Indices=5  OutputSizes=1
  Selector4 : Selector  InputPortWidth=8  IndexOptions=Index vector (dialog)  Indices=4  OutputSizes=1
  Selector5 : Selector  InputPortWidth=8  IndexOptions=Index vector (dialog)  Indices=3  OutputSizes=1
  Selector6 : Selector  InputPortWidth=8  IndexOptions=Index vector (dialog)  Indices=2  OutputSizes=1
  Selector7 : Selector  InputPortWidth=8  IndexOptions=Index vector (dialog)  Indices=1  OutputSizes=1
  SSR : Outport
  wires:
  Bit Concat/1 -> SSR/1
  Vector/1 -> Selector0/1, Selector1/1, Selector2/1, Selector3/1, Selector4/1, Selector5/1, Selector6/1, Selector7/1
  Selector0/1 -> Bit Concat/1
  Selector1/1 -> Bit Concat/2
  Selector2/1 -> Bit Concat/3
  Selector3/1 -> Bit Concat/4
  Selector4/1 -> Bit Concat/5
  Selector5/1 -> Bit Concat/6
  Selector6/1 -> Bit Concat/7
  Selector7/1 -> Bit Concat/8

== system demonstrator/FINNadapter/Decimation/Stimulus and Channel/Channel/RF-DAC/NCO and Mixer/RF-DAC Coarse Mixer ==
  Data In : Inport
  Add2 : Sum  OutDataTypeStr=double
  Complex to Real-Imag : ComplexToRealImag
  Constant : Constant  Value=mc  OutDataTypeStr=fixdt(0,2,0)  SampleTime=-1
  Multiport Switch1 : MultiPortSwitch  DataPortOrder=Zero-based contiguous  zeroidx=on
  Negate : Subsystem
  fs_2 : Subsystem
  fs_4 : Subsystem
  Data Out : Outport  VectorParamsAs1DForOutWhenUnconnected=off
  wires:
  fs_4/1(Data Out) -> Multiport Switch1/3, Negate/1(Data In)
  Negate/1(Data Out) -> Multiport Switch1/4
  Data In/1 -> fs_2/1(Data In), fs_4/1(Data In)
  Constant/1 -> Multiport Switch1/1
  fs_2/1(Data Out) -> Multiport Switch1/2
  Multiport Switch1/1 -> Complex to Real-Imag/1
  Complex to Real-Imag/1 -> Add2/1
  Complex to Real-Imag/2 -> Add2/2
  Add2/1 -> Data Out/1

== system demonstrator/FINNadapter/Decimation/Stimulus and Channel/Channel/RF-DAC/NCO and Mixer/RF-DAC Fine Mixer ==
  Data In : Inport
  Add2 : Sum
  Complex to Real-Imag1 : ComplexToRealImag
  Constant : Constant  OutDataTypeStr=boolean  SampleTime=-1
  Multiport Switch : MultiPortSwitch  DataPortOrder=Zero-based contiguous  Inputs=2  zeroidx=on
  NCO : dspsigops/NCO  AccIncSrc=Specify via dialog  AccInc=fix((((fc*1e9)*(2^18))/(fs))*2^30)  PhaseOffsetSrc=Specify via dialog  PhaseOffset=fix((((2^18)*fph)/(2*pi))*2^30)  AccumWL=48  HasDither=off  DitherWL=4  PNgeneratorLength=19  HasPhaseQuantizer=on  TableDepth=18  HasOutputPhaseError=off  Formula=Sine and cosine  DataType=Binary point scaling  OutputWL=16  OutputFL=15  CompMethod=Table lookup (no interpolation)  SampleTime=1/(fs)  SamplesPerFrame=ssr  OutputFrames=off
      settings: SourceProductBaseCode=DS
  Product1 : Product
  Product4 : Product
  Shift Arithmetic1 : ArithShift  BitShiftNumber=1  BitShiftDirection=Right
  Data Out : Outport  VectorParamsAs1DForOutWhenUnconnected=off
  wires:
  Shift Arithmetic1/1 -> Multiport Switch/3
  Add2/1 -> Multiport Switch/2, Shift Arithmetic1/1
  Multiport Switch/1 -> Data Out/1
  Constant/1 -> Multiport Switch/1
  Data In/1 -> Complex to Real-Imag1/1
  Product4/1 -> Add2/1
  NCO/1 -> Product4/2
  Complex to Real-Imag1/2 -> Product4/1
  Product1/1 -> Add2/2
  Complex to Real-Imag1/1 -> Product1/1
  NCO/2 -> Product1/2

== system demonstrator/FINNadapter/Decimation/Stimulus and Channel/Channel/RF-DAC/SSR Converter RF-DAC/SSR to Vector Low ==
  SSR : Inport
  Bit Slice0 : hdlsllib/Logic and Bit Operations/Bit Slice  lidx=31  ridx=0
      settings: SourceProductBaseCode=SL
  Bit Slice1 : hdlsllib/Logic and Bit Operations/Bit Slice  lidx=63  ridx=32
      settings: SourceProductBaseCode=SL
  Bit Slice2 : hdlsllib/Logic and Bit Operations/Bit Slice  lidx=95  ridx=64
      settings: SourceProductBaseCode=SL
  Bit Slice3 : hdlsllib/Logic and Bit Operations/Bit Slice  lidx=127  ridx=96
      settings: SourceProductBaseCode=SL
  Matrix Concatenate : Concatenate  NumInputs=4  Mode=Multidimensional array
  Vector : Outport
  wires:
  Matrix Concatenate/1 -> Vector/1
  SSR/1 -> Bit Slice0/1, Bit Slice1/1, Bit Slice2/1, Bit Slice3/1
  Bit Slice0/1 -> Matrix Concatenate/1
  Bit Slice1/1 -> Matrix Concatenate/2
  Bit Slice2/1 -> Matrix Concatenate/3
  Bit Slice3/1 -> Matrix Concatenate/4

== system demonstrator/FINNadapter/Decimation/Stimulus and Channel/Channel/RF-ADC/NCO and Mixer/RF-ADC Coarse Mixer/Negate ==
  Data In : Inport
  Complex to Real-Imag2 : ComplexToRealImag
  Real-Imag to Complex1 : RealImagToComplex
  Unary Minus : UnaryMinus
  Data Out : Outport  VectorParamsAs1DForOutWhenUnconnected=off
  wires:
  Complex to Real-Imag2/2 -> Unary Minus/1
  Unary Minus/1 -> Real-Imag to Complex1/2
  Data In/1 -> Complex to Real-Imag2/1
  Real-Imag to Complex1/1 -> Data Out/1
  Complex to Real-Imag2/1 -> Real-Imag to Complex1/1
